simulink model "pwm_code_gen"  (R2017b)
settings: Solver=FixedStepDiscrete  StartTime=0.0  StopTime=10000*T  FixedStep=T  RelTol=1e-3
InitFcn:
  | T = 1/50e6;
libraries: simulink x1
settings Model: Creator=roman  LastModifiedBy=roman

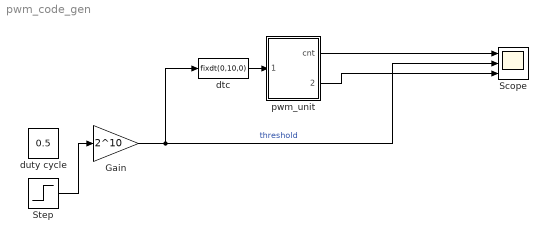
== system pwm_code_gen ==
  Gain : Gain  Gain=2^10
  Scope : Scope  NumInputPorts=3
  Step : Step  Time=5000*T  Before=0.5  After=0.7  SampleTime=0
  dtc : DataTypeConversion  OutDataTypeStr=fixdt(0,10,0)
  duty cycle : Constant  Value=0.5
  pwm_unit : Subsystem
  wires:
  Gain/1 -> dtc/1, Scope/2  "threshold"
  Step/1 -> Gain/1
  pwm_unit/1(cnt) -> Scope/1
  pwm_unit/2(pwm) -> Scope/3
  dtc/1 -> pwm_unit/1(threshold)

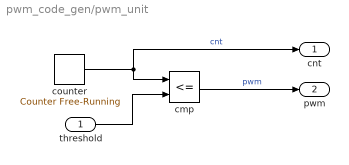
== system pwm_code_gen/pwm_unit ==
  threshold : Inport
  cmp : RelationalOperator  Operator=<=  OutDataTypeStr=boolean  RndMeth=Simplest
  counter : simulink/Sources/Counter Free-Running  NumBits=10  tsamp=-1
  cnt : Outport
  pwm : Outport  Port=2
  wires:
  counter/1 -> cnt/1, cmp/1  "cnt"
  cmp/1 -> pwm/1  "pwm"
  threshold/1 -> cmp/2
